simulink model "u2pwm"  (R2016b)
settings: Solver=ode3  StartTime=0.0  StopTime=inf  FixedStep=0.01  RelTol=1e-3  EnableMultiTasking=on
values from neighbouring files (symbols this model uses):
  alpha_rate_limit = 2*360/(60*s_scaled)    [initfile.m]
  Max_thrust = 1.5    [initfile.m]
  Min_thrust = -0.8    [initfile.m]
  pwm_thr1_backward = coeffvalues(ForceToPWM)    [initfile.m]
  pwm_thr1_forward = coeffvalues(ForceToPWM)    [initfile.m]
  pwm_thr2_backward = coeffvalues(ForceToPWM)    [initfile.m]
  pwm_thr2_forward = coeffvalues(ForceToPWM)    [initfile.m]
  pwm_thr3_backward = coeffvalues(ForceToPWM)    [initfile.m]
  pwm_thr3_forward = coeffvalues(ForceToPWM)    [initfile.m]
  pwm_thr4_backward = coeffvalues(ForceToPWM)    [initfile.m]
  pwm_thr4_forward = coeffvalues(ForceToPWM)    [initfile.m]
  pwm_thr5_backward = coeffvalues(ForceToPWM)    [initfile.m]
  pwm_thr5_forward = coeffvalues(ForceToPWM)    [initfile.m]
  pwm_thr6_backward = coeffvalues(ForceToPWM)    [initfile.m]
  pwm_thr6_forward = coeffvalues(ForceToPWM)    [initfile.m]
  zero_alpha_1 = -90    [initfile.m]
  zero_alpha_2 = -40    [initfile.m]
  zero_alpha_3 = 5    [initfile.m]
  zero_alpha_4 = -25    [initfile.m]
  zero_alpha_5 = 127    [initfile.m]
  zero_alpha_6 = -34    [initfile.m]
  zero_pwm = min_pwm + u2pwm_gain    (= 7.5)    [initfile.m]
(part 3 of 3)

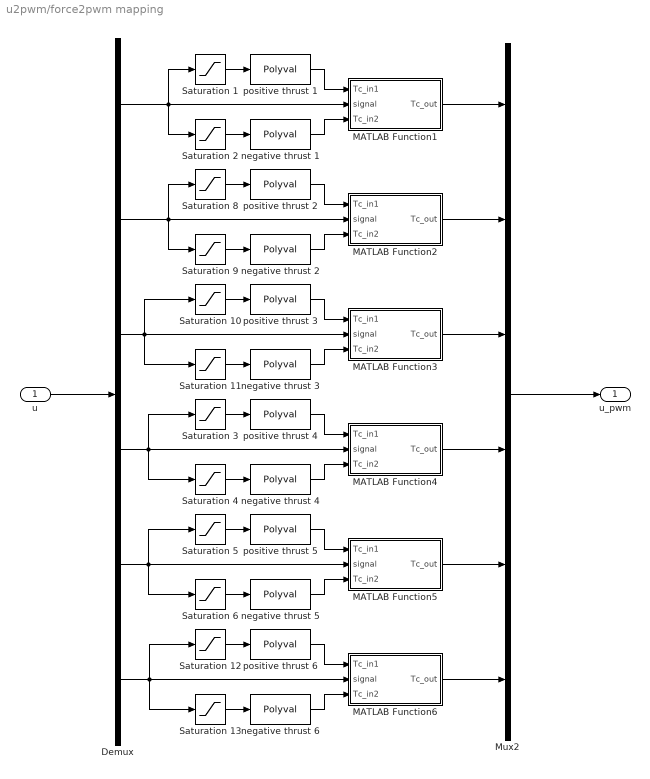
== system u2pwm/force2pwm mapping ==
  u : Inport
  Demux : Demux  Outputs=6
  MATLAB Function1 : MATLAB Function  TreatAsAtomicUnit=on
  MATLAB Function2 : MATLAB Function  TreatAsAtomicUnit=on
  MATLAB Function3 : MATLAB Function  TreatAsAtomicUnit=on
  MATLAB Function4 : MATLAB Function  TreatAsAtomicUnit=on
  MATLAB Function5 : MATLAB Function  TreatAsAtomicUnit=on
  MATLAB Function6 : MATLAB Function  TreatAsAtomicUnit=on
  Mux2 : Mux  Inputs=6
  Saturation {1,3,5,8,10,12} (6 alike) : Saturate  UpperLimit=Max_thrust  LowerLimit=0
  Saturation {2,4,6,9,11,13} (6 alike) : Saturate  UpperLimit=0  LowerLimit=Min_thrust
  negative thrust 1 : Polyval  Coefs=pwm_thr1_backward
  negative thrust 2 : Polyval  Coefs=pwm_thr2_backward
  negative thrust 3 : Polyval  Coefs=pwm_thr3_backward
  negative thrust 4 : Polyval  Coefs=pwm_thr4_backward
  negative thrust 5 : Polyval  Coefs=pwm_thr5_backward
  negative thrust 6 : Polyval  Coefs=pwm_thr6_backward
  positive thrust 1 : Polyval  Coefs=pwm_thr1_forward
  positive thrust 2 : Polyval  Coefs=pwm_thr2_forward
  positive thrust 3 : Polyval  Coefs=pwm_thr3_forward
  positive thrust 4 : Polyval  Coefs=pwm_thr4_forward
  positive thrust 5 : Polyval  Coefs=pwm_thr5_forward
  positive thrust 6 : Polyval  Coefs=pwm_thr6_forward
  u_pwm : Outport
  wires:
  Mux2/1 -> u_pwm/1
  u/1 -> Demux/1
  Saturation 2/1 -> negative thrust 1/1
  positive thrust 2/1 -> MATLAB Function2/1(Tc_in1)
  Demux/1 -> Saturation 1/1, MATLAB Function1/2(signal), Saturation 2/1
  MATLAB Function1/1(Tc_out) -> Mux2/1
  Saturation 8/1 -> positive thrust 2/1
  Saturation 11/1 -> negative thrust 3/1
  MATLAB Function4/1(Tc_out) -> Mux2/4
  positive thrust 3/1 -> MATLAB Function3/1(Tc_in1)
  Demux/3 -> Saturation 11/1, MATLAB Function3/2(signal), Saturation 10/1
  Saturation 3/1 -> positive thrust 4/1
  Saturation 4/1 -> negative thrust 4/1
  positive thrust 5/1 -> MATLAB Function5/1(Tc_in1)
  negative thrust 5/1 -> MATLAB Function5/3(Tc_in2)
  MATLAB Function5/1(Tc_out) -> Mux2/5
  Saturation 5/1 -> positive thrust 5/1
  Demux/5 -> Saturation 5/1, MATLAB Function5/2(signal), Saturation 6/1
  negative thrust 1/1 -> MATLAB Function1/3(Tc_in2)
  negative thrust 2/1 -> MATLAB Function2/3(Tc_in2)
  Saturation 6/1 -> negative thrust 5/1
  negative thrust 6/1 -> MATLAB Function6/3(Tc_in2)
  MATLAB Function3/1(Tc_out) -> Mux2/3
  positive thrust 6/1 -> MATLAB Function6/1(Tc_in1)
  negative thrust 3/1 -> MATLAB Function3/3(Tc_in2)
  Saturation 1/1 -> positive thrust 1/1
  MATLAB Function2/1(Tc_out) -> Mux2/2
  Saturation 9/1 -> negative thrust 2/1
  Demux/2 -> Saturation 9/1, Saturation 8/1, MATLAB Function2/2(signal)
  Saturation 10/1 -> positive thrust 3/1
  positive thrust 4/1 -> MATLAB Function4/1(Tc_in1)
  negative thrust 4/1 -> MATLAB Function4/3(Tc_in2)
  Demux/4 -> Saturation 3/1, Saturation 4/1, MATLAB Function4/2(signal)
  positive thrust 1/1 -> MATLAB Function1/1(Tc_in1)
  MATLAB Function6/1(Tc_out) -> Mux2/6
  Saturation 12/1 -> positive thrust 6/1
  Demux/6 -> Saturation 13/1, Saturation 12/1, MATLAB Function6/2(signal)
  Saturation 13/1 -> negative thrust 6/1

== system u2pwm/indicator ==
  switch_signal : Inport
  C : MATLAB Function  TreatAsAtomicUnit=on
  STOP : S-Function  Priority=1  FunctionName=NIVeriStandIO  Parameters=width dtype portnum stime stype btype  SFunctionDeploymentMode=off  EnableBusSupport=off  mask(NI VeriStand Outport){portnum=1, width=-1, stime=-1, dtype=auto, stype=auto, btype=0}
      mask prompts: portnum "Port number:"; width "Port dimensions (-1 for dynamically sized):"; stime "Sample time (-1 for inherited):"; dtype "Data type:"; stype "Signal type:"; btype "Block type:"
      mask help: Use this outport on any level of nested subsystems to allow NI VeriStand software to map signals to it.
      mask init:
      | NIVeriStandIO_init;
      settings: CopyFcn=NIVeriStand_MDL_functions('', 'IO_copy');  DeleteFcn=NIVeriStand_MDL_functions('', 'IO_delete');  MoveFcn=set_param(gcb, 'Mask', 'on');
      mask Callback portnum: NIVeriStand_MDL_functions('', 'IO_setportnum');
      mask TypeOptions dtype: auto | double | single | int8 | uint8 | int16 | uint16 | int32 | uint32 | boolean
      mask Callback dtype: NIVeriStand_MDL_functions('', 'IO_booleansignal');
      mask TypeOptions stype: auto | real | complex
      mask Display:
      | patch([-x x], [-y y], [.90980 .81960 .32156]);
      | plot([xrad -x x xrad], [yrad -y y yrad]);
      | fprintf('NI Out%d', portnum);
  ctrl_DP : S-Function  Priority=2  FunctionName=NIVeriStandIO  Parameters=width dtype portnum stime stype btype  SFunctionDeploymentMode=off  EnableBusSupport=off  mask(NI VeriStand Outport){portnum=2, width=-1, stime=-1, dtype=auto, stype=auto, btype=0}
      mask prompts: portnum "Port number:"; width "Port dimensions (-1 for dynamically sized):"; stime "Sample time (-1 for inherited):"; dtype "Data type:"; stype "Signal type:"; btype "Block type:"
      mask help: Use this outport on any level of nested subsystems to allow NI VeriStand software to map signals to it.
      mask init:
      | NIVeriStandIO_init;
      settings: CopyFcn=NIVeriStand_MDL_functions('', 'IO_copy');  DeleteFcn=NIVeriStand_MDL_functions('', 'IO_delete');  MoveFcn=set_param(gcb, 'Mask', 'on');
      mask Callback portnum: NIVeriStand_MDL_functions('', 'IO_setportnum');
      mask TypeOptions dtype: auto | double | single | int8 | uint8 | int16 | uint16 | int32 | uint32 | boolean
      mask Callback dtype: NIVeriStand_MDL_functions('', 'IO_booleansignal');
      mask TypeOptions stype: auto | real | complex
      mask Display:
      | patch([-x x], [-y y], [.90980 .81960 .32156]);
      | plot([xrad -x x xrad], [yrad -y y yrad]);
      | fprintf('NI Out%d', portnum);
  ctrl_custom : S-Function  Priority=4  FunctionName=NIVeriStandIO  Parameters=width dtype portnum stime stype btype  SFunctionDeploymentMode=off  EnableBusSupport=off  mask(NI VeriStand Outport){portnum=4, width=-1, stime=-1, dtype=auto, stype=auto, btype=0}
      mask prompts: portnum "Port number:"; width "Port dimensions (-1 for dynamically sized):"; stime "Sample time (-1 for inherited):"; dtype "Data type:"; stype "Signal type:"; btype "Block type:"
      mask help: Use this outport on any level of nested subsystems to allow NI VeriStand software to map signals to it.
      mask init:
      | NIVeriStandIO_init;
      settings: CopyFcn=NIVeriStand_MDL_functions('', 'IO_copy');  DeleteFcn=NIVeriStand_MDL_functions('', 'IO_delete');  MoveFcn=set_param(gcb, 'Mask', 'on');
      mask Callback portnum: NIVeriStand_MDL_functions('', 'IO_setportnum');
      mask TypeOptions dtype: auto | double | single | int8 | uint8 | int16 | uint16 | int32 | uint32 | boolean
      mask Callback dtype: NIVeriStand_MDL_functions('', 'IO_booleansignal');
      mask TypeOptions stype: auto | real | complex
      mask Display:
      | patch([-x x], [-y y], [.90980 .81960 .32156]);
      | plot([xrad -x x xrad], [yrad -y y yrad]);
      | fprintf('NI Out%d', portnum);
  ctrl_sixaxis2thruster : S-Function  Priority=3  FunctionName=NIVeriStandIO  Parameters=width dtype portnum stime stype btype  SFunctionDeploymentMode=off  EnableBusSupport=off  mask(NI VeriStand Outport){portnum=3, width=-1, stime=-1, dtype=auto, stype=auto, btype=0}
      mask prompts: portnum "Port number:"; width "Port dimensions (-1 for dynamically sized):"; stime "Sample time (-1 for inherited):"; dtype "Data type:"; stype "Signal type:"; btype "Block type:"
      mask help: Use this outport on any level of nested subsystems to allow NI VeriStand software to map signals to it.
      mask init:
      | NIVeriStandIO_init;
      settings: CopyFcn=NIVeriStand_MDL_functions('', 'IO_copy');  DeleteFcn=NIVeriStand_MDL_functions('', 'IO_delete');  MoveFcn=set_param(gcb, 'Mask', 'on');
      mask Callback portnum: NIVeriStand_MDL_functions('', 'IO_setportnum');
      mask TypeOptions dtype: auto | double | single | int8 | uint8 | int16 | uint16 | int32 | uint32 | boolean
      mask Callback dtype: NIVeriStand_MDL_functions('', 'IO_booleansignal');
      mask TypeOptions stype: auto | real | complex
      mask Display:
      | patch([-x x], [-y y], [.90980 .81960 .32156]);
      | plot([xrad -x x xrad], [yrad -y y yrad]);
      | fprintf('NI Out%d', portnum);
  wires:
  switch_signal/1 -> C/1(switch_signal)
  C/4(ctrl_sixaxis2thruster) -> ctrl_sixaxis2thruster/1
  C/3(ctrl_DP) -> ctrl_DP/1
  C/2(STOP) -> STOP/1
  C/1(ctrl_custom) -> ctrl_custom/1

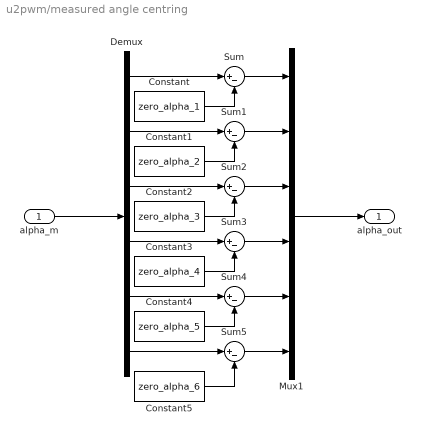
== system u2pwm/measured angle centring ==
  alpha_m : Inport
  Constant : Constant  Value=zero_alpha_1
  Constant1 : Constant  Value=zero_alpha_2
  Constant2 : Constant  Value=zero_alpha_3
  Constant3 : Constant  Value=zero_alpha_4
  Constant4 : Constant  Value=zero_alpha_5
  Constant5 : Constant  Value=zero_alpha_6
  Demux : Demux  Outputs=6
  Mux1 : Mux  Inputs=6
  Sum{,1..5} (6 alike) : Sum  Inputs=|+-
  alpha_out : Outport
  wires:
  Mux1/1 -> alpha_out/1
  alpha_m/1 -> Demux/1
  Constant4/1 -> Sum4/2
  Demux/4 -> Sum3/1
  Constant1/1 -> Sum1/2
  Demux/2 -> Sum1/1
  Demux/1 -> Sum/1
  Constant/1 -> Sum/2
  Constant2/1 -> Sum2/2
  Constant3/1 -> Sum3/2
  Demux/5 -> Sum4/1
  Demux/3 -> Sum2/1
  Demux/6 -> Sum5/1
  Constant5/1 -> Sum5/2
  Sum5/1 -> Mux1/6
  Sum3/1 -> Mux1/4
  Sum/1 -> Mux1/1
  Sum2/1 -> Mux1/3
  Sum1/1 -> Mux1/2
  Sum4/1 -> Mux1/5

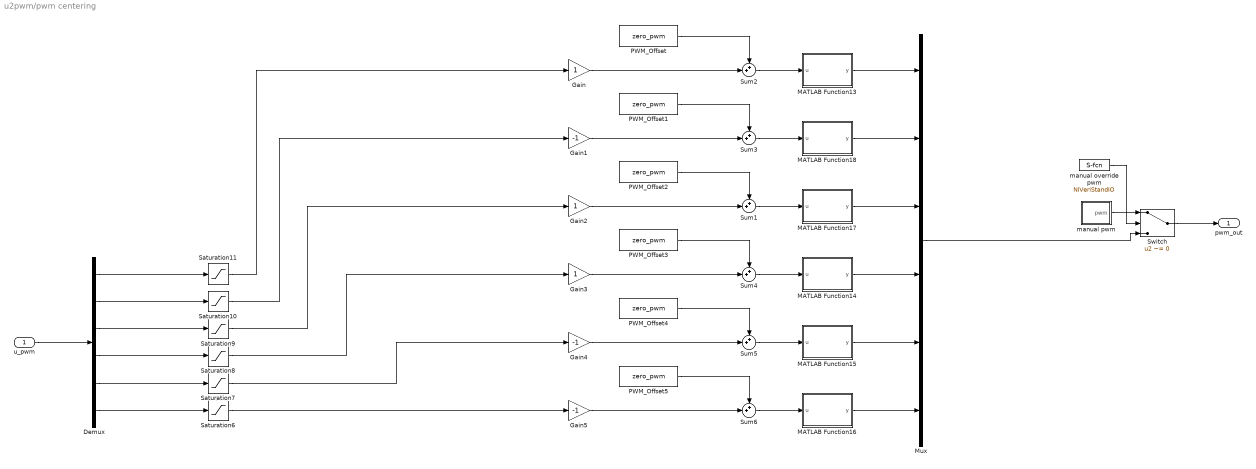
== system u2pwm/pwm centering ==
  u_pwm : Inport
  Demux : Demux  Outputs=6
  Gain : Gain
  Gain1 : Gain  Gain=-1
  Gain2 : Gain
  Gain3 : Gain
  Gain4 : Gain  Gain=-1
  Gain5 : Gain  Gain=-1
  MATLAB Function13 : MATLAB Function  TreatAsAtomicUnit=on
  MATLAB Function14 : MATLAB Function  TreatAsAtomicUnit=on
  MATLAB Function15 : MATLAB Function  TreatAsAtomicUnit=on
  MATLAB Function16 : MATLAB Function  TreatAsAtomicUnit=on
  MATLAB Function17 : MATLAB Function  TreatAsAtomicUnit=on
  MATLAB Function18 : MATLAB Function  TreatAsAtomicUnit=on
  Mux : Mux  Inputs=6
  PWM_Offset{,1..5} (6 alike) : Constant  Value=zero_pwm
  Saturation{6..11} (6 alike) : Saturate
  Sum{1..6} (6 alike) : Sum  Inputs=++|
  Switch : Switch  Criteria=u2 ~= 0
  manual override pwm : S-Function  Priority=9  FunctionName=NIVeriStandIO  Parameters=width dtype portnum stime stype btype  SFunctionDeploymentMode=off  EnableBusSupport=off  mask(NI VeriStand Inport){portnum=9, width=-1, stime=-1, dtype=auto, stype=auto, btype=1}
      mask prompts: portnum "Port number:"; width "Port dimensions (-1 for dynamically sized):"; stime "Sample time (-1 for inherited):"; dtype "Data type:"; stype "Signal type:"; btype "Block type:"
      mask help: Use this inport on any level of nested subsystems to allow NI VeriStand software to map signals to it.
      mask init:
      | NIVeriStandIO_init;
      settings: CopyFcn=NIVeriStand_MDL_functions('', 'IO_copy');  DeleteFcn=NIVeriStand_MDL_functions('', 'IO_delete');  MoveFcn=set_param(gcb, 'Mask', 'on');
      mask Callback portnum: NIVeriStand_MDL_functions('', 'IO_setportnum');
      mask TypeOptions dtype: auto | double | single | int8 | uint8 | int16 | uint16 | int32 | uint32 | boolean
      mask Callback dtype: NIVeriStand_MDL_functions('', 'IO_booleansignal');
      mask TypeOptions stype: auto | real | complex
      mask Display:
      | patch([-x x], [-y y], [.90980 .81960 .32156]);
      | plot([xrad -x x xrad], [yrad -y y yrad]);
      | fprintf('NI In%d', portnum);
  manual pwm : Subsystem
  pwm_out : Outport
  wires:
  u_pwm/1 -> Demux/1
  Saturation6/1 -> Gain5/1
  MATLAB Function16/1(y) -> Mux/6
  MATLAB Function15/1(y) -> Mux/5
  MATLAB Function14/1(y) -> Mux/4
  MATLAB Function17/1(y) -> Mux/3
  MATLAB Function18/1(y) -> Mux/2
  MATLAB Function13/1(y) -> Mux/1
  Sum6/1 -> MATLAB Function16/1(u)
  Sum5/1 -> MATLAB Function15/1(u)
  Sum4/1 -> MATLAB Function14/1(u)
  Sum1/1 -> MATLAB Function17/1(u)
  Sum3/1 -> MATLAB Function18/1(u)
  Sum2/1 -> MATLAB Function13/1(u)
  PWM_Offset4/1 -> Sum5/1
  Saturation7/1 -> Gain4/1
  Gain5/1 -> Sum6/2
  PWM_Offset5/1 -> Sum6/1
  Mux/1 -> Switch/3
  Saturation9/1 -> Gain2/1
  manual pwm/1(pwm) -> Switch/1
  PWM_Offset1/1 -> Sum3/1
  PWM_Offset2/1 -> Sum1/1
  Gain2/1 -> Sum1/2
  Saturation10/1 -> Gain1/1
  Gain1/1 -> Sum3/2
  manual override pwm/1 -> Switch/2
  Gain/1 -> Sum2/2
  Switch/1 -> pwm_out/1
  Saturation11/1 -> Gain/1
  PWM_Offset/1 -> Sum2/1
  Saturation8/1 -> Gain3/1
  Gain3/1 -> Sum4/2
  PWM_Offset3/1 -> Sum4/1
  Gain4/1 -> Sum5/2
  Demux/1 -> Saturation11/1
  Demux/2 -> Saturation10/1
  Demux/3 -> Saturation9/1
  Demux/4 -> Saturation8/1
  Demux/5 -> Saturation7/1
  Demux/6 -> Saturation6/1

== system u2pwm/pwm_output u ==
  pwm : Inport
  Demux1 : Demux  Outputs=6
  pwm_u_1 : S-Function  Priority=3  FunctionName=NIVeriStandIO  Parameters=width dtype portnum stime stype btype  SFunctionDeploymentMode=off  EnableBusSupport=off  mask(NI VeriStand Outport){portnum=3, width=-1, stime=-1, dtype=auto, stype=auto, btype=0}
      mask prompts: portnum "Port number:"; width "Port dimensions (-1 for dynamically sized):"; stime "Sample time (-1 for inherited):"; dtype "Data type:"; stype "Signal type:"; btype "Block type:"
      mask help: Use this outport on any level of nested subsystems to allow NI VeriStand software to map signals to it.
      mask init:
      | NIVeriStandIO_init;
      settings: CopyFcn=NIVeriStand_MDL_functions('', 'IO_copy');  DeleteFcn=NIVeriStand_MDL_functions('', 'IO_delete');  MoveFcn=set_param(gcb, 'Mask', 'on');
      mask Callback portnum: NIVeriStand_MDL_functions('', 'IO_setportnum');
      mask TypeOptions dtype: auto | double | single | int8 | uint8 | int16 | uint16 | int32 | uint32 | boolean
      mask Callback dtype: NIVeriStand_MDL_functions('', 'IO_booleansignal');
      mask TypeOptions stype: auto | real | complex
      mask Display:
      | patch([-x x], [-y y], [.90980 .81960 .32156]);
      | plot([xrad -x x xrad], [yrad -y y yrad]);
      | fprintf('NI Out%d', portnum);
  pwm_u_2 : S-Function  Priority=1  FunctionName=NIVeriStandIO  Parameters=width dtype portnum stime stype btype  SFunctionDeploymentMode=off  EnableBusSupport=off  mask(NI VeriStand Outport){portnum=1, width=-1, stime=-1, dtype=auto, stype=auto, btype=0}
      mask prompts: portnum "Port number:"; width "Port dimensions (-1 for dynamically sized):"; stime "Sample time (-1 for inherited):"; dtype "Data type:"; stype "Signal type:"; btype "Block type:"
      mask help: Use this outport on any level of nested subsystems to allow NI VeriStand software to map signals to it.
      mask init:
      | NIVeriStandIO_init;
      settings: CopyFcn=NIVeriStand_MDL_functions('', 'IO_copy');  DeleteFcn=NIVeriStand_MDL_functions('', 'IO_delete');  MoveFcn=set_param(gcb, 'Mask', 'on');
      mask Callback portnum: NIVeriStand_MDL_functions('', 'IO_setportnum');
      mask TypeOptions dtype: auto | double | single | int8 | uint8 | int16 | uint16 | int32 | uint32 | boolean
      mask Callback dtype: NIVeriStand_MDL_functions('', 'IO_booleansignal');
      mask TypeOptions stype: auto | real | complex
      mask Display:
      | patch([-x x], [-y y], [.90980 .81960 .32156]);
      | plot([xrad -x x xrad], [yrad -y y yrad]);
      | fprintf('NI Out%d', portnum);
  pwm_u_3 : S-Function  Priority=2  FunctionName=NIVeriStandIO  Parameters=width dtype portnum stime stype btype  SFunctionDeploymentMode=off  EnableBusSupport=off  mask(NI VeriStand Outport){portnum=2, width=-1, stime=-1, dtype=auto, stype=auto, btype=0}
      mask prompts: portnum "Port number:"; width "Port dimensions (-1 for dynamically sized):"; stime "Sample time (-1 for inherited):"; dtype "Data type:"; stype "Signal type:"; btype "Block type:"
      mask help: Use this outport on any level of nested subsystems to allow NI VeriStand software to map signals to it.
      mask init:
      | NIVeriStandIO_init;
      settings: CopyFcn=NIVeriStand_MDL_functions('', 'IO_copy');  DeleteFcn=NIVeriStand_MDL_functions('', 'IO_delete');  MoveFcn=set_param(gcb, 'Mask', 'on');
      mask Callback portnum: NIVeriStand_MDL_functions('', 'IO_setportnum');
      mask TypeOptions dtype: auto | double | single | int8 | uint8 | int16 | uint16 | int32 | uint32 | boolean
      mask Callback dtype: NIVeriStand_MDL_functions('', 'IO_booleansignal');
      mask TypeOptions stype: auto | real | complex
      mask Display:
      | patch([-x x], [-y y], [.90980 .81960 .32156]);
      | plot([xrad -x x xrad], [yrad -y y yrad]);
      | fprintf('NI Out%d', portnum);
  pwm_u_4 : S-Function  Priority=5  FunctionName=NIVeriStandIO  Parameters=width dtype portnum stime stype btype  SFunctionDeploymentMode=off  EnableBusSupport=off  mask(NI VeriStand Outport){portnum=5, width=-1, stime=-1, dtype=auto, stype=auto, btype=0}
      mask prompts: portnum "Port number:"; width "Port dimensions (-1 for dynamically sized):"; stime "Sample time (-1 for inherited):"; dtype "Data type:"; stype "Signal type:"; btype "Block type:"
      mask help: Use this outport on any level of nested subsystems to allow NI VeriStand software to map signals to it.
      mask init:
      | NIVeriStandIO_init;
      settings: CopyFcn=NIVeriStand_MDL_functions('', 'IO_copy');  DeleteFcn=NIVeriStand_MDL_functions('', 'IO_delete');  MoveFcn=set_param(gcb, 'Mask', 'on');
      mask Callback portnum: NIVeriStand_MDL_functions('', 'IO_setportnum');
      mask TypeOptions dtype: auto | double | single | int8 | uint8 | int16 | uint16 | int32 | uint32 | boolean
      mask Callback dtype: NIVeriStand_MDL_functions('', 'IO_booleansignal');
      mask TypeOptions stype: auto | real | complex
      mask Display:
      | patch([-x x], [-y y], [.90980 .81960 .32156]);
      | plot([xrad -x x xrad], [yrad -y y yrad]);
      | fprintf('NI Out%d', portnum);
  pwm_u_5 : S-Function  Priority=6  FunctionName=NIVeriStandIO  Parameters=width dtype portnum stime stype btype  SFunctionDeploymentMode=off  EnableBusSupport=off  mask(NI VeriStand Outport){portnum=6, width=-1, stime=-1, dtype=auto, stype=auto, btype=0}
      mask prompts: portnum "Port number:"; width "Port dimensions (-1 for dynamically sized):"; stime "Sample time (-1 for inherited):"; dtype "Data type:"; stype "Signal type:"; btype "Block type:"
      mask help: Use this outport on any level of nested subsystems to allow NI VeriStand software to map signals to it.
      mask init:
      | NIVeriStandIO_init;
      settings: CopyFcn=NIVeriStand_MDL_functions('', 'IO_copy');  DeleteFcn=NIVeriStand_MDL_functions('', 'IO_delete');  MoveFcn=set_param(gcb, 'Mask', 'on');
      mask Callback portnum: NIVeriStand_MDL_functions('', 'IO_setportnum');
      mask TypeOptions dtype: auto | double | single | int8 | uint8 | int16 | uint16 | int32 | uint32 | boolean
      mask Callback dtype: NIVeriStand_MDL_functions('', 'IO_booleansignal');
      mask TypeOptions stype: auto | real | complex
      mask Display:
      | patch([-x x], [-y y], [.90980 .81960 .32156]);
      | plot([xrad -x x xrad], [yrad -y y yrad]);
      | fprintf('NI Out%d', portnum);
  pwm_u_6 : S-Function  Priority=4  FunctionName=NIVeriStandIO  Parameters=width dtype portnum stime stype btype  SFunctionDeploymentMode=off  EnableBusSupport=off  mask(NI VeriStand Outport){portnum=4, width=-1, stime=-1, dtype=auto, stype=auto, btype=0}
      mask prompts: portnum "Port number:"; width "Port dimensions (-1 for dynamically sized):"; stime "Sample time (-1 for inherited):"; dtype "Data type:"; stype "Signal type:"; btype "Block type:"
      mask help: Use this outport on any level of nested subsystems to allow NI VeriStand software to map signals to it.
      mask init:
      | NIVeriStandIO_init;
      settings: CopyFcn=NIVeriStand_MDL_functions('', 'IO_copy');  DeleteFcn=NIVeriStand_MDL_functions('', 'IO_delete');  MoveFcn=set_param(gcb, 'Mask', 'on');
      mask Callback portnum: NIVeriStand_MDL_functions('', 'IO_setportnum');
      mask TypeOptions dtype: auto | double | single | int8 | uint8 | int16 | uint16 | int32 | uint32 | boolean
      mask Callback dtype: NIVeriStand_MDL_functions('', 'IO_booleansignal');
      mask TypeOptions stype: auto | real | complex
      mask Display:
      | patch([-x x], [-y y], [.90980 .81960 .32156]);
      | plot([xrad -x x xrad], [yrad -y y yrad]);
      | fprintf('NI Out%d', portnum);
  wires:
  Demux1/1 -> pwm_u_1/1
  Demux1/3 -> pwm_u_3/1
  Demux1/5 -> pwm_u_5/1
  Demux1/6 -> pwm_u_6/1
  Demux1/2 -> pwm_u_2/1
  Demux1/4 -> pwm_u_4/1
  pwm/1 -> Demux1/1

== system u2pwm/rate constrainer ==
  alpha : Inport
  Integrator : Integrator  InitialCondition=[0 0 0 0 0 0]'
  Saturation : Saturate  UpperLimit=alpha_rate_limit  LowerLimit=-alpha_rate_limit
  Sum : Sum  Inputs=|+-
  alpha_out : Outport
  wires:
  Integrator/1 -> alpha_out/1, Sum/2
  alpha/1 -> Sum/1
  Sum/1 -> Saturation/1
  Saturation/1 -> Integrator/1

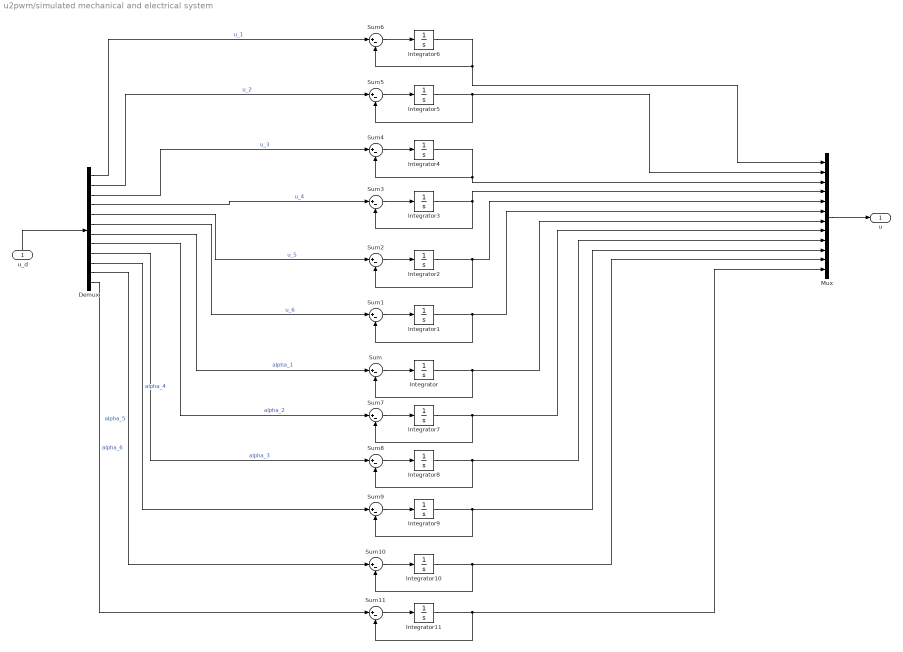
== system u2pwm/simulated mechanical and electrical system ==
  u_d : Inport
  Demux : Demux  Outputs=12
  Integrator{,1..11} (12 alike) : Integrator
  Mux : Mux  Inputs=12
  Sum{,1..11} (12 alike) : Sum  Inputs=|+-
  u : Outport
  wires:
  Demux/6 -> Sum1/1  "u_6"
  Demux/3 -> Sum4/1  "u_3"
  Demux/2 -> Sum5/1  "u_2"
  Demux/4 -> Sum3/1  "u_4"
  Demux/5 -> Sum2/1  "u_5"
  Demux/7 -> Sum/1  "alpha_1"
  Demux/1 -> Sum6/1  "u_1"
  u_d/1 -> Demux/1
  Mux/1 -> u/1
  Sum/1 -> Integrator/1
  Integrator/1 -> Sum/2, Mux/7
  Sum1/1 -> Integrator1/1
  Integrator1/1 -> Sum1/2, Mux/6
  Sum2/1 -> Integrator2/1
  Integrator2/1 -> Sum2/2, Mux/5
  Sum3/1 -> Integrator3/1
  Integrator3/1 -> Sum3/2, Mux/4
  Sum4/1 -> Integrator4/1
  Integrator4/1 -> Mux/3, Sum4/2
  Sum5/1 -> Integrator5/1
  Integrator5/1 -> Sum5/2, Mux/2
  Sum6/1 -> Integrator6/1
  Integrator6/1 -> Sum6/2, Mux/1
  Demux/8 -> Sum7/1  "alpha_2"
  Sum7/1 -> Integrator7/1
  Integrator7/1 -> Mux/8, Sum7/2
  Demux/9 -> Sum8/1  "alpha_3"
  Sum8/1 -> Integrator8/1
  Integrator8/1 -> Mux/9, Sum8/2
  Demux/10 -> Sum9/1  "alpha_4"
  Sum9/1 -> Integrator9/1
  Integrator9/1 -> Mux/10, Sum9/2
  Demux/11 -> Sum10/1  "alpha_5"
  Sum10/1 -> Integrator10/1
  Integrator10/1 -> Mux/11, Sum10/2
  Demux/12 -> Sum11/1  "alpha_6"
  Sum11/1 -> Integrator11/1
  Integrator11/1 -> Mux/12, Sum11/2

== system u2pwm/angle centering/manual alpha ==
  Mux : Mux  Inputs=6
  man_alpha_1 : S-Function  Priority=3  FunctionName=NIVeriStandIO  Parameters=width dtype portnum stime stype btype  SFunctionDeploymentMode=off  EnableBusSupport=off  mask(NI VeriStand Inport){portnum=3, width=-1, stime=-1, dtype=auto, stype=auto, btype=1}
      mask prompts: portnum "Port number:"; width "Port dimensions (-1 for dynamically sized):"; stime "Sample time (-1 for inherited):"; dtype "Data type:"; stype "Signal type:"; btype "Block type:"
      mask help: Use this inport on any level of nested subsystems to allow NI VeriStand software to map signals to it.
      mask init:
      | NIVeriStandIO_init;
      settings: CopyFcn=NIVeriStand_MDL_functions('', 'IO_copy');  DeleteFcn=NIVeriStand_MDL_functions('', 'IO_delete');  MoveFcn=set_param(gcb, 'Mask', 'on');
      mask Callback portnum: NIVeriStand_MDL_functions('', 'IO_setportnum');
      mask TypeOptions dtype: auto | double | single | int8 | uint8 | int16 | uint16 | int32 | uint32 | boolean
      mask Callback dtype: NIVeriStand_MDL_functions('', 'IO_booleansignal');
      mask TypeOptions stype: auto | real | complex
      mask Display:
      | patch([-x x], [-y y], [.90980 .81960 .32156]);
      | plot([xrad -x x xrad], [yrad -y y yrad]);
      | fprintf('NI In%d', portnum);
  man_alpha_2 : S-Function  Priority=4  FunctionName=NIVeriStandIO  Parameters=width dtype portnum stime stype btype  SFunctionDeploymentMode=off  EnableBusSupport=off  mask(NI VeriStand Inport){portnum=4, width=-1, stime=-1, dtype=auto, stype=auto, btype=1}
      mask prompts: portnum "Port number:"; width "Port dimensions (-1 for dynamically sized):"; stime "Sample time (-1 for inherited):"; dtype "Data type:"; stype "Signal type:"; btype "Block type:"
      mask help: Use this inport on any level of nested subsystems to allow NI VeriStand software to map signals to it.
      mask init:
      | NIVeriStandIO_init;
      settings: CopyFcn=NIVeriStand_MDL_functions('', 'IO_copy');  DeleteFcn=NIVeriStand_MDL_functions('', 'IO_delete');  MoveFcn=set_param(gcb, 'Mask', 'on');
      mask Callback portnum: NIVeriStand_MDL_functions('', 'IO_setportnum');
      mask TypeOptions dtype: auto | double | single | int8 | uint8 | int16 | uint16 | int32 | uint32 | boolean
      mask Callback dtype: NIVeriStand_MDL_functions('', 'IO_booleansignal');
      mask TypeOptions stype: auto | real | complex
      mask Display:
      | patch([-x x], [-y y], [.90980 .81960 .32156]);
      | plot([xrad -x x xrad], [yrad -y y yrad]);
      | fprintf('NI In%d', portnum);
  man_alpha_3 : S-Function  Priority=5  FunctionName=NIVeriStandIO  Parameters=width dtype portnum stime stype btype  SFunctionDeploymentMode=off  EnableBusSupport=off  mask(NI VeriStand Inport){portnum=5, width=-1, stime=-1, dtype=auto, stype=auto, btype=1}
      mask prompts: portnum "Port number:"; width "Port dimensions (-1 for dynamically sized):"; stime "Sample time (-1 for inherited):"; dtype "Data type:"; stype "Signal type:"; btype "Block type:"
      mask help: Use this inport on any level of nested subsystems to allow NI VeriStand software to map signals to it.
      mask init:
      | NIVeriStandIO_init;
      settings: CopyFcn=NIVeriStand_MDL_functions('', 'IO_copy');  DeleteFcn=NIVeriStand_MDL_functions('', 'IO_delete');  MoveFcn=set_param(gcb, 'Mask', 'on');
      mask Callback portnum: NIVeriStand_MDL_functions('', 'IO_setportnum');
      mask TypeOptions dtype: auto | double | single | int8 | uint8 | int16 | uint16 | int32 | uint32 | boolean
      mask Callback dtype: NIVeriStand_MDL_functions('', 'IO_booleansignal');
      mask TypeOptions stype: auto | real | complex
      mask Display:
      | patch([-x x], [-y y], [.90980 .81960 .32156]);
      | plot([xrad -x x xrad], [yrad -y y yrad]);
      | fprintf('NI In%d', portnum);
  man_alpha_4 : S-Function  Priority=2  FunctionName=NIVeriStandIO  Parameters=width dtype portnum stime stype btype  SFunctionDeploymentMode=off  EnableBusSupport=off  mask(NI VeriStand Inport){portnum=2, width=-1, stime=-1, dtype=auto, stype=auto, btype=1}
      mask prompts: portnum "Port number:"; width "Port dimensions (-1 for dynamically sized):"; stime "Sample time (-1 for inherited):"; dtype "Data type:"; stype "Signal type:"; btype "Block type:"
      mask help: Use this inport on any level of nested subsystems to allow NI VeriStand software to map signals to it.
      mask init:
      | NIVeriStandIO_init;
      settings: CopyFcn=NIVeriStand_MDL_functions('', 'IO_copy');  DeleteFcn=NIVeriStand_MDL_functions('', 'IO_delete');  MoveFcn=set_param(gcb, 'Mask', 'on');
      mask Callback portnum: NIVeriStand_MDL_functions('', 'IO_setportnum');
      mask TypeOptions dtype: auto | double | single | int8 | uint8 | int16 | uint16 | int32 | uint32 | boolean
      mask Callback dtype: NIVeriStand_MDL_functions('', 'IO_booleansignal');
      mask TypeOptions stype: auto | real | complex
      mask Display:
      | patch([-x x], [-y y], [.90980 .81960 .32156]);
      | plot([xrad -x x xrad], [yrad -y y yrad]);
      | fprintf('NI In%d', portnum);
  man_alpha_5 : S-Function  Priority=1  FunctionName=NIVeriStandIO  Parameters=width dtype portnum stime stype btype  SFunctionDeploymentMode=off  EnableBusSupport=off  mask(NI VeriStand Inport){portnum=1, width=-1, stime=-1, dtype=auto, stype=auto, btype=1}
      mask prompts: portnum "Port number:"; width "Port dimensions (-1 for dynamically sized):"; stime "Sample time (-1 for inherited):"; dtype "Data type:"; stype "Signal type:"; btype "Block type:"
      mask help: Use this inport on any level of nested subsystems to allow NI VeriStand software to map signals to it.
      mask init:
      | NIVeriStandIO_init;
      settings: CopyFcn=NIVeriStand_MDL_functions('', 'IO_copy');  DeleteFcn=NIVeriStand_MDL_functions('', 'IO_delete');  MoveFcn=set_param(gcb, 'Mask', 'on');
      mask Callback portnum: NIVeriStand_MDL_functions('', 'IO_setportnum');
      mask TypeOptions dtype: auto | double | single | int8 | uint8 | int16 | uint16 | int32 | uint32 | boolean
      mask Callback dtype: NIVeriStand_MDL_functions('', 'IO_booleansignal');
      mask TypeOptions stype: auto | real | complex
      mask Display:
      | patch([-x x], [-y y], [.90980 .81960 .32156]);
      | plot([xrad -x x xrad], [yrad -y y yrad]);
      | fprintf('NI In%d', portnum);
  man_alpha_6 : S-Function  Priority=6  FunctionName=NIVeriStandIO  Parameters=width dtype portnum stime stype btype  SFunctionDeploymentMode=off  EnableBusSupport=off  mask(NI VeriStand Inport){portnum=6, width=-1, stime=-1, dtype=auto, stype=auto, btype=1}
      mask prompts: portnum "Port number:"; width "Port dimensions (-1 for dynamically sized):"; stime "Sample time (-1 for inherited):"; dtype "Data type:"; stype "Signal type:"; btype "Block type:"
      mask help: Use this inport on any level of nested subsystems to allow NI VeriStand software to map signals to it.
      mask init:
      | NIVeriStandIO_init;
      settings: CopyFcn=NIVeriStand_MDL_functions('', 'IO_copy');  DeleteFcn=NIVeriStand_MDL_functions('', 'IO_delete');  MoveFcn=set_param(gcb, 'Mask', 'on');
      mask Callback portnum: NIVeriStand_MDL_functions('', 'IO_setportnum');
      mask TypeOptions dtype: auto | double | single | int8 | uint8 | int16 | uint16 | int32 | uint32 | boolean
      mask Callback dtype: NIVeriStand_MDL_functions('', 'IO_booleansignal');
      mask TypeOptions stype: auto | real | complex
      mask Display:
      | patch([-x x], [-y y], [.90980 .81960 .32156]);
      | plot([xrad -x x xrad], [yrad -y y yrad]);
      | fprintf('NI In%d', portnum);
  alpha : Outport
  wires:
  man_alpha_1/1 -> Mux/1
  man_alpha_6/1 -> Mux/6
  man_alpha_2/1 -> Mux/2
  man_alpha_4/1 -> Mux/4
  man_alpha_5/1 -> Mux/5
  Mux/1 -> alpha/1
  man_alpha_3/1 -> Mux/3

== system u2pwm/pwm centering/manual pwm ==
  Mux : Mux  Inputs=6
  pwm_u_1 : S-Function  Priority=3  FunctionName=NIVeriStandIO  Parameters=width dtype portnum stime stype btype  SFunctionDeploymentMode=off  EnableBusSupport=off  mask(NI VeriStand Inport){portnum=3, width=-1, stime=-1, dtype=auto, stype=auto, btype=1}
      mask prompts: portnum "Port number:"; width "Port dimensions (-1 for dynamically sized):"; stime "Sample time (-1 for inherited):"; dtype "Data type:"; stype "Signal type:"; btype "Block type:"
      mask help: Use this inport on any level of nested subsystems to allow NI VeriStand software to map signals to it.
      mask init:
      | NIVeriStandIO_init;
      settings: CopyFcn=NIVeriStand_MDL_functions('', 'IO_copy');  DeleteFcn=NIVeriStand_MDL_functions('', 'IO_delete');  MoveFcn=set_param(gcb, 'Mask', 'on');
      mask Callback portnum: NIVeriStand_MDL_functions('', 'IO_setportnum');
      mask TypeOptions dtype: auto | double | single | int8 | uint8 | int16 | uint16 | int32 | uint32 | boolean
      mask Callback dtype: NIVeriStand_MDL_functions('', 'IO_booleansignal');
      mask TypeOptions stype: auto | real | complex
      mask Display:
      | patch([-x x], [-y y], [.90980 .81960 .32156]);
      | plot([xrad -x x xrad], [yrad -y y yrad]);
      | fprintf('NI In%d', portnum);
  pwm_u_2 : S-Function  Priority=5  FunctionName=NIVeriStandIO  Parameters=width dtype portnum stime stype btype  SFunctionDeploymentMode=off  EnableBusSupport=off  mask(NI VeriStand Inport){portnum=5, width=-1, stime=-1, dtype=auto, stype=auto, btype=1}
      mask prompts: portnum "Port number:"; width "Port dimensions (-1 for dynamically sized):"; stime "Sample time (-1 for inherited):"; dtype "Data type:"; stype "Signal type:"; btype "Block type:"
      mask help: Use this inport on any level of nested subsystems to allow NI VeriStand software to map signals to it.
      mask init:
      | NIVeriStandIO_init;
      settings: CopyFcn=NIVeriStand_MDL_functions('', 'IO_copy');  DeleteFcn=NIVeriStand_MDL_functions('', 'IO_delete');  MoveFcn=set_param(gcb, 'Mask', 'on');
      mask Callback portnum: NIVeriStand_MDL_functions('', 'IO_setportnum');
      mask TypeOptions dtype: auto | double | single | int8 | uint8 | int16 | uint16 | int32 | uint32 | boolean
      mask Callback dtype: NIVeriStand_MDL_functions('', 'IO_booleansignal');
      mask TypeOptions stype: auto | real | complex
      mask Display:
      | patch([-x x], [-y y], [.90980 .81960 .32156]);
      | plot([xrad -x x xrad], [yrad -y y yrad]);
      | fprintf('NI In%d', portnum);
  pwm_u_3 : S-Function  Priority=6  FunctionName=NIVeriStandIO  Parameters=width dtype portnum stime stype btype  SFunctionDeploymentMode=off  EnableBusSupport=off  mask(NI VeriStand Inport){portnum=6, width=-1, stime=-1, dtype=auto, stype=auto, btype=1}
      mask prompts: portnum "Port number:"; width "Port dimensions (-1 for dynamically sized):"; stime "Sample time (-1 for inherited):"; dtype "Data type:"; stype "Signal type:"; btype "Block type:"
      mask help: Use this inport on any level of nested subsystems to allow NI VeriStand software to map signals to it.
      mask init:
      | NIVeriStandIO_init;
      settings: CopyFcn=NIVeriStand_MDL_functions('', 'IO_copy');  DeleteFcn=NIVeriStand_MDL_functions('', 'IO_delete');  MoveFcn=set_param(gcb, 'Mask', 'on');
      mask Callback portnum: NIVeriStand_MDL_functions('', 'IO_setportnum');
      mask TypeOptions dtype: auto | double | single | int8 | uint8 | int16 | uint16 | int32 | uint32 | boolean
      mask Callback dtype: NIVeriStand_MDL_functions('', 'IO_booleansignal');
      mask TypeOptions stype: auto | real | complex
      mask Display:
      | patch([-x x], [-y y], [.90980 .81960 .32156]);
      | plot([xrad -x x xrad], [yrad -y y yrad]);
      | fprintf('NI In%d', portnum);
  pwm_u_4 : S-Function  Priority=2  FunctionName=NIVeriStandIO  Parameters=width dtype portnum stime stype btype  SFunctionDeploymentMode=off  EnableBusSupport=off  mask(NI VeriStand Inport){portnum=2, width=-1, stime=-1, dtype=auto, stype=auto, btype=1}
      mask prompts: portnum "Port number:"; width "Port dimensions (-1 for dynamically sized):"; stime "Sample time (-1 for inherited):"; dtype "Data type:"; stype "Signal type:"; btype "Block type:"
      mask help: Use this inport on any level of nested subsystems to allow NI VeriStand software to map signals to it.
      mask init:
      | NIVeriStandIO_init;
      settings: CopyFcn=NIVeriStand_MDL_functions('', 'IO_copy');  DeleteFcn=NIVeriStand_MDL_functions('', 'IO_delete');  MoveFcn=set_param(gcb, 'Mask', 'on');
      mask Callback portnum: NIVeriStand_MDL_functions('', 'IO_setportnum');
      mask TypeOptions dtype: auto | double | single | int8 | uint8 | int16 | uint16 | int32 | uint32 | boolean
      mask Callback dtype: NIVeriStand_MDL_functions('', 'IO_booleansignal');
      mask TypeOptions stype: auto | real | complex
      mask Display:
      | patch([-x x], [-y y], [.90980 .81960 .32156]);
      | plot([xrad -x x xrad], [yrad -y y yrad]);
      | fprintf('NI In%d', portnum);
  pwm_u_5 : S-Function  Priority=1  FunctionName=NIVeriStandIO  Parameters=width dtype portnum stime stype btype  SFunctionDeploymentMode=off  EnableBusSupport=off  mask(NI VeriStand Inport){portnum=1, width=-1, stime=-1, dtype=auto, stype=auto, btype=1}
      mask prompts: portnum "Port number:"; width "Port dimensions (-1 for dynamically sized):"; stime "Sample time (-1 for inherited):"; dtype "Data type:"; stype "Signal type:"; btype "Block type:"
      mask help: Use this inport on any level of nested subsystems to allow NI VeriStand software to map signals to it.
      mask init:
      | NIVeriStandIO_init;
      settings: CopyFcn=NIVeriStand_MDL_functions('', 'IO_copy');  DeleteFcn=NIVeriStand_MDL_functions('', 'IO_delete');  MoveFcn=set_param(gcb, 'Mask', 'on');
      mask Callback portnum: NIVeriStand_MDL_functions('', 'IO_setportnum');
      mask TypeOptions dtype: auto | double | single | int8 | uint8 | int16 | uint16 | int32 | uint32 | boolean
      mask Callback dtype: NIVeriStand_MDL_functions('', 'IO_booleansignal');
      mask TypeOptions stype: auto | real | complex
      mask Display:
      | patch([-x x], [-y y], [.90980 .81960 .32156]);
      | plot([xrad -x x xrad], [yrad -y y yrad]);
      | fprintf('NI In%d', portnum);
  pwm_u_6 : S-Function  Priority=4  FunctionName=NIVeriStandIO  Parameters=width dtype portnum stime stype btype  SFunctionDeploymentMode=off  EnableBusSupport=off  mask(NI VeriStand Inport){portnum=4, width=-1, stime=-1, dtype=auto, stype=auto, btype=1}
      mask prompts: portnum "Port number:"; width "Port dimensions (-1 for dynamically sized):"; stime "Sample time (-1 for inherited):"; dtype "Data type:"; stype "Signal type:"; btype "Block type:"
      mask help: Use this inport on any level of nested subsystems to allow NI VeriStand software to map signals to it.
      mask init:
      | NIVeriStandIO_init;
      settings: CopyFcn=NIVeriStand_MDL_functions('', 'IO_copy');  DeleteFcn=NIVeriStand_MDL_functions('', 'IO_delete');  MoveFcn=set_param(gcb, 'Mask', 'on');
      mask Callback portnum: NIVeriStand_MDL_functions('', 'IO_setportnum');
      mask TypeOptions dtype: auto | double | single | int8 | uint8 | int16 | uint16 | int32 | uint32 | boolean
      mask Callback dtype: NIVeriStand_MDL_functions('', 'IO_booleansignal');
      mask TypeOptions stype: auto | real | complex
      mask Display:
      | patch([-x x], [-y y], [.90980 .81960 .32156]);
      | plot([xrad -x x xrad], [yrad -y y yrad]);
      | fprintf('NI In%d', portnum);
  pwm : Outport
  wires:
  pwm_u_1/1 -> Mux/1
  pwm_u_6/1 -> Mux/6
  pwm_u_2/1 -> Mux/2
  pwm_u_4/1 -> Mux/4
  pwm_u_5/1 -> Mux/5
  Mux/1 -> pwm/1
  pwm_u_3/1 -> Mux/3

== matlab function u2pwm/indicator/C ==
  data: switch_signal input; ctrl_custom output; STOP output; ctrl_DP output; ctrl_sixaxis2thruster output
function [ctrl_custom,STOP,ctrl_DP,ctrl_sixaxis2thruster]= fcn(switch_signal)

ctrl_sixaxis2thruster = false;
ctrl_DP    = false;
STOP         = false;
ctrl_custom          = false;

if switch_signal     == 1
    ctrl_custom          = true; 
elseif switch_signal == 2
    ctrl_DP    = true; 
elseif switch_signal == 3
    STOP         = true; 
elseif switch_signal == 4
    ctrl_sixaxis2thruster = true;
else
    
end

== matlab function u2pwm/Switch_subsystem/Switch_function ==
  data: Cross input; switch_signal output; Square input; Circle input; Triangle input; temp input
%% Function that takes in impulse button sigals [0,1] and sends out a 
% different signal depentent pn which button has been pressed

function switch_signal = fcn(Cross,Square,Circle,Triangle,temp)
%#codegen
persistent signal;

signal = temp;

if Cross ~= 0
    signal = 1;
end

if Square ~= 0
    signal = 2;
end

if Circle ~= 0
    signal = 3;
end
    
if Triangle ~= 0
    signal = 4; 
end

switch_signal = signal;

== matlab function u2pwm/control limit checking ==
  data: u input; fault output
function fault= fcn(u)
u_1     = u(1);
u_2     = u(2);
u_3     = u(3);
u_4     = u(4);
u_5     = u(5);
u_6     = u(6);

OK = -1   <= u_1        & u_1        <= 1  & ...
     -1   <= u_2        & u_2        <= 1  & ...
     -1   <= u_3        & u_3        <= 1  & ...
     -1   <= u_4        & u_4        <= 1  & ...
     -1   <= u_5        & u_5        <= 1  & ...
     -1   <= u_6        & u_6        <= 1;
 
fault = ~OK;

== matlab function u2pwm/MATLAB Function ==
  data: alpha_m_step input; alpha_m_deg output
function alpha_m_deg = step2deg(alpha_m_step)

puls = 32768; 
degpp = 23002/puls; %Degrees pr. pulse.
% positionData = uint32(positionData); %Convert from double to uint32

%Convertion to signed data:
counterNBits = 15; %Bits in the encoder reading
signedThreshold = 2^(counterNBits-1); %Treshold for convertion to signed pos. values
signedData = alpha_m_step;
signedData(signedData > signedThreshold) = signedData(signedData > signedThreshold) - 2^counterNBits;

alpha_m_deg = signedData*degpp;

end

== matlab function u2pwm/angle centering/Exceeding max angle test ==
  data: u input; y output
function y = fcn(u)

max_angle = 9000;

if u(1) > 3200 || u(1) < -max_angle
    y = 1;
elseif u(2) > max_angle || u(2) < -max_angle
    y = 1;
elseif u(3) > max_angle || u(3) < -max_angle
    y = 1;
elseif u(4) > max_angle || u(4) < -max_angle
    y = 1;
elseif u(5) > max_angle || u(5) < -max_angle
    y = 1;
elseif u(6) > max_angle || u(6) < -max_angle
    y = 1;
else 
    y = 0;
end


end

== matlab function u2pwm/pwm centering/MATLAB Function13 ==
  data: u input; y output
function y = fcn(u)

if u == 7.5
    y = u;
elseif u < 7.5
    y = u - 0.31;
else
    y = u + 0.31;
end

end

== matlab function u2pwm/pwm centering/MATLAB Function14 ==
  data: u input; y output
function y = fcn(u)

if u == 7.5
    y = u;
elseif u < 7.5
    y = u - 0.31;
else
    y = u + 0.31;
end

end

== matlab function u2pwm/pwm centering/MATLAB Function15 ==
  data: u input; y output
function y = fcn(u)

if u == 7.5
    y = u;
elseif u < 7.5
    y = u - 0.31;
else
    y = u + 0.31;
end

end

== matlab function u2pwm/pwm centering/MATLAB Function16 ==
  data: u input; y output
function y = fcn(u)

if u == 7.5
    y = u;
elseif u < 7.5
    y = u - 0.31;
else
    y = u + 0.31;
end

end

== matlab function u2pwm/pwm centering/MATLAB Function17 ==
  data: u input; y output
function y = fcn(u)

if u == 7.5
    y = u;
elseif u < 7.5
    y = u - 0.31;
else
    y = u + 0.31;
end

end

== matlab function u2pwm/pwm centering/MATLAB Function18 ==
  data: u input; y output
function y = fcn(u)

if u == 7.5
    y = u;
elseif u < 7.5
    y = u - 0.31;
else
    y = u + 0.31;
end

end

== matlab function u2pwm/force2pwm mapping/MATLAB Function1 ==
  data: Tc_in1 input; signal input; Tc_out output; Tc_in2 input
function Tc_out = fcn(Tc_in1,signal,Tc_in2)
%#codegen

if signal >= 0
    Tc_out = Tc_in1;
else %signal < 0
    Tc_out = Tc_in2;
end

== matlab function u2pwm/force2pwm mapping/MATLAB Function2 ==
  data: Tc_in1 input; signal input; Tc_out output; Tc_in2 input
function Tc_out = fcn(Tc_in1,signal,Tc_in2)
%#codegen

if signal >= 0
    Tc_out = Tc_in1;
else %signal < 0
    Tc_out = Tc_in2;
end

== matlab function u2pwm/force2pwm mapping/MATLAB Function3 ==
  data: Tc_in1 input; signal input; Tc_out output; Tc_in2 input
function Tc_out = fcn(Tc_in1,signal,Tc_in2)
%#codegen

if signal >= 0
    Tc_out = Tc_in1;
else %signal < 0
    Tc_out = Tc_in2;
end

== matlab function u2pwm/force2pwm mapping/MATLAB Function4 ==
  data: Tc_in1 input; signal input; Tc_out output; Tc_in2 input
function Tc_out = fcn(Tc_in1,signal,Tc_in2)
%#codegen

if signal >= 0
    Tc_out = Tc_in1;
else %signal < 0
    Tc_out = Tc_in2;
end

== matlab function u2pwm/force2pwm mapping/MATLAB Function5 ==
  data: Tc_in1 input; signal input; Tc_out output; Tc_in2 input
function Tc_out = fcn(Tc_in1,signal,Tc_in2)
%#codegen

if signal >= 0
    Tc_out = Tc_in1;
else %signal < 0
    Tc_out = Tc_in2;
end

== matlab function u2pwm/force2pwm mapping/MATLAB Function6 ==
  data: Tc_in1 input; signal input; Tc_out output; Tc_in2 input
function Tc_out = fcn(Tc_in1,signal,Tc_in2)
%#codegen

if signal >= 0
    Tc_out = Tc_in1;
else %signal < 0
    Tc_out = Tc_in2;
end
